simulink model "p2d1"  (R2023b)
settings: Solver=VariableStepAuto  StartTime=0.0  StopTime=10.0  RelTol=1e-3
settings Model: Creator=tanvi  LastModifiedBy=tanvi

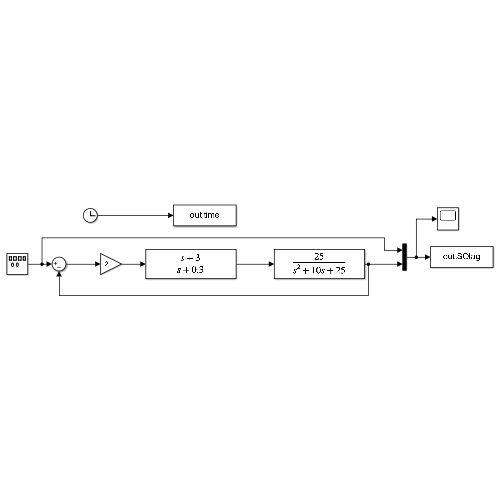
[thumbnail: Simulink's stored preview of the top-level diagram]
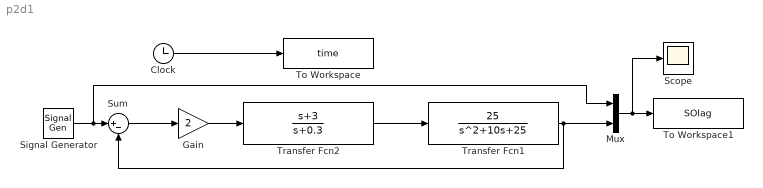
== system p2d1 ==
  Clock : Clock
  Gain : Gain  Gain=2
  Mux : Mux  Inputs=2
  Scope : Scope
  Signal Generator : SignalGenerator  WaveForm=square  Frequency=0.15
  Sum : Sum  Inputs=|+-
  To Workspace : ToWorkspace  VariableName=time  SampleTime=-1
  To Workspace1 : ToWorkspace  VariableName=SOlag  SampleTime=-1
  Transfer Fcn1 : TransferFcn  Numerator=[25]  Denominator=[1 10 25]
  Transfer Fcn2 : TransferFcn  Numerator=[1 3]  Denominator=[1 0.3]
  wires:
  Gain/1 -> Transfer Fcn2/1
  Transfer Fcn2/1 -> Transfer Fcn1/1
  Sum/1 -> Gain/1
  Signal Generator/1 -> Mux/1, Sum/1
  Clock/1 -> To Workspace/1
  Mux/1 -> To Workspace1/1, Scope/1
  Transfer Fcn1/1 -> Sum/2, Mux/2
